simulink model "tiaofu"  (R2020b)
settings: Solver=VariableStepAuto  StartTime=0.0  StopTime=1  RelTol=1e-3
libraries: dsparch4 x1
settings Model: Creator=QinKai  LastModifiedBy=QinKai

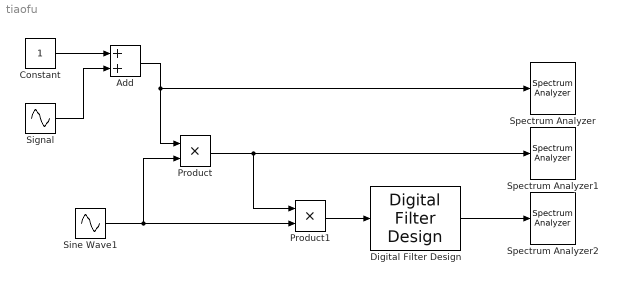
== system tiaofu ==
  Add : Sum
  Constant : Constant
  Digital Filter Design : dsparch4/Digital Filter Design  mwdsp_browser_bugfix_var=off
  Product : Product
  Product1 : Product
  Signal : Sin  Frequency=2*pi*1e3  SampleTime=1/24e3
  Sine Wave1 : Sin  Amplitude=2  Frequency=2*pi*4e3  SampleTime=1/24e3
  Spectrum Analyzer : SpectrumAnalyzer
  Spectrum Analyzer1 : SpectrumAnalyzer
  Spectrum Analyzer2 : SpectrumAnalyzer
  wires:
  Sine Wave1/1 -> Product1/2, Product/2
  Product/1 -> Spectrum Analyzer1/1, Product1/1
  Product1/1 -> Digital Filter Design/1
  Digital Filter Design/1 -> Spectrum Analyzer2/1
  Add/1 -> Spectrum Analyzer/1, Product/1
  Constant/1 -> Add/1
  Signal/1 -> Add/2
